simulink model "MIP_LQGcontroller"  (R2020b)
settings: Solver=VariableStepAuto  StartTime=0.0  StopTime=5  RelTol=1e-3
values from neighbouring files (symbols this model uses):
  A = [-(a+b)*j*XX (a+b)*j*XX a*d*XX;(b+c)*j*XX -(b+c)*j*XX -b*d*XX;1 0 0]    [Parameters.m]
  B = [-(a+b)*e*XX; (b+c)*e*XX; 0]    [Parameters.m]
  C = [1 0 0;0 1 0;0 0 1]    [Parameters.m]
  Cy_all = [0 1 0;0 1 0;0 0 1]    [LQG_controller.m]
  Cy_phidot = [0 1 0]    [LQG_controller.m]
  Cy_phidot_theta = [0 1 0;0 0 1]    [LQG_controller.m]
  Cy_theta = [0 0 1]    [LQG_controller.m]
  Cy_thetadot = [1 0 0]    [LQG_controller.m]
  Cy_thetadot_phidot = [1 0 0;0 1 0]    [LQG_controller.m]
  Cy_thetadot_theta = [1 0 0;0 0 1]    [LQG_controller.m]
  D = [0;0;0]    [Parameters.m]
  F_all = -F'    [LQG_controller.m]
  F_phidot = -F'    [LQG_controller.m]
  F_phidot_theta = -F'    [LQG_controller.m]
  F_theta = -F'    [LQG_controller.m]
  F_thetadot = -F'    [LQG_controller.m]
  F_thetadot_phidot = -F'    [LQG_controller.m]
  F_thetadot_theta = -F'    [LQG_controller.m]
  K_all = -K    [LQG_controller.m]
  K_phidot = -K    [LQG_controller.m]
  K_phidot_theta = -K    [LQG_controller.m]
  K_theta = -K    [LQG_controller.m]
  K_thetadot = -K    [LQG_controller.m]
  K_thetadot_phidot = -K    [LQG_controller.m]
  K_thetadot_theta = -K    [LQG_controller.m]
  V_max = 7.4    [Parameters.m]
settings Model: Creator=arthur  LastModifiedBy=arthur

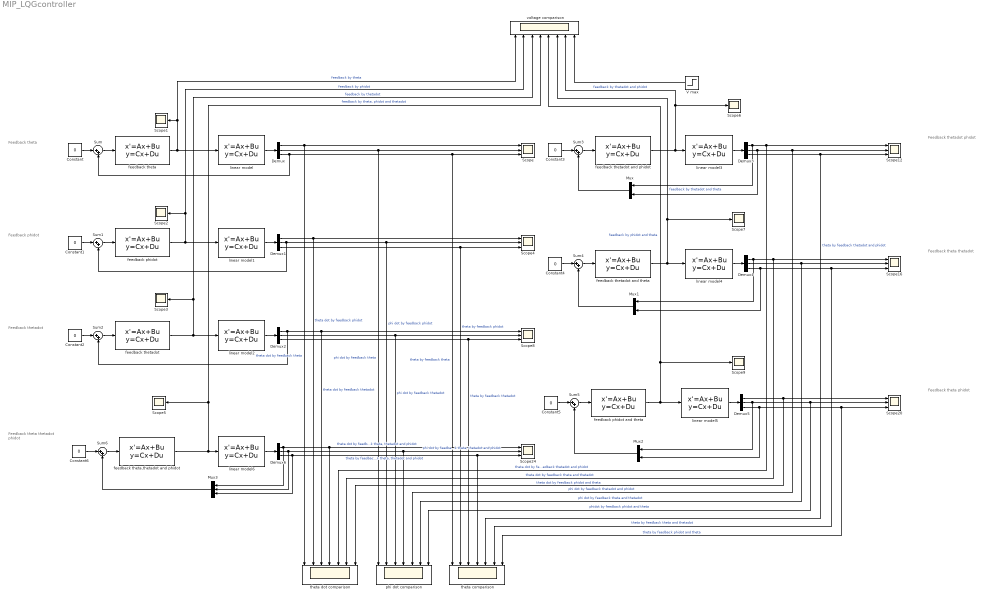
== system MIP_LQGcontroller ==
  note: Feedback
      | theta
  note: Feedback
      | phidot
  note: Feedback
      | thetadot
  note: Feedback
      | theta
      | thetadot
      | phidot
  note: Feedback
      | thetadot
      | phidot
  note: Feedback
      | theta
      | thetadot
  note: Feedback
      | theta
      | phidot
  Constant{,1..6} (7 alike) : Constant  Value=0
  Demux{,1..6} (7 alike) : Demux  Outputs=3
  Mux : Mux  Inputs=2
  Mux1 : Mux  Inputs=2
  Mux2 : Mux  Inputs=2
  Mux3 : Mux  Inputs=3
  Scope{,4,8,12,16,20,24} (7 alike) : Scope  NumInputPorts=3
  Scope{1..3,5..7,9} (7 alike) : Scope
  Sum{,1..6} (7 alike) : Sum  Inputs=|++
  V max : Step  Time=0  After=V_max  SampleTime=0
  feedback phidot : StateSpace  A=A+B*K_phidot+F_phidot*Cy_phidot  B=-F_phidot  C=K_phidot  D=0  InitialCondition=0
  feedback phidot and theta : StateSpace  A=A+B*K_phidot_theta+F_phidot_theta*Cy_phidot_theta  B=-F_phidot_theta  C=K_phidot_theta  D=[0 0]  InitialCondition=0
  feedback theta : StateSpace  A=A+B*K_theta+F_theta*Cy_theta  B=-F_theta  C=K_theta  D=0  InitialCondition=0
  feedback theta,thetadot and phidot : StateSpace  A=A+B*K_all+F_all*Cy_all  B=-F_all  C=K_all  D=[0 0 0]  InitialCondition=0
  feedback thetadot : StateSpace  A=A+B*K_thetadot+F_thetadot*Cy_thetadot  B=-F_thetadot  C=K_thetadot  D=0  InitialCondition=0
  feedback thetadot and phidot : StateSpace  A=A+B*K_thetadot_phidot+F_thetadot_phidot*Cy_thetadot_phidot  B=-F_thetadot_phidot  C=K_thetadot_phidot  D=[0 0]  InitialCondition=0
  feedback thetadot and theta : StateSpace  A=A+B*K_thetadot_theta+F_thetadot_theta*Cy_thetadot_theta  B=-F_thetadot_theta  C=K_thetadot_theta  D=[0 0]  InitialCondition=0
  linear model : StateSpace  A=A  B=B  C=C  D=D  InitialCondition=[0 0 49*pi/180]
  linear model1 : StateSpace  A=A  B=B  C=C  D=D  InitialCondition=[0 0 29*pi/180]
  linear model2 : StateSpace  A=A  B=B  C=C  D=D  InitialCondition=[0 0 30*pi/180]
  linear model3 : StateSpace  A=A  B=B  C=C  D=D  InitialCondition=[0 0 56*pi/180]
  linear model4 : StateSpace  A=A  B=B  C=C  D=D  InitialCondition=[0 0 74*pi/180]
  linear model5 : StateSpace  A=A  B=B  C=C  D=D  InitialCondition=[0 0 48*pi/180]
  linear model6 : StateSpace  A=A  B=B  C=C  D=D  InitialCondition=[0 0 43*pi/180]
  phi dot comparison : Scope  NumInputPorts=7
  theta comparison : Scope  NumInputPorts=7
  theta dot comparison : Scope  NumInputPorts=7
  voltage comparison : Scope  NumInputPorts=8
  wires:
  linear model/1 -> Demux/1
  Demux/1 -> Scope/1, theta dot comparison/1  "theta dot by feedback theta"
  Demux/3 -> Sum/2, Scope/3, theta comparison/1  "theta by feedback theta"
  feedback theta/1 -> linear model/1, Scope1/1, voltage comparison/1  "feedback by theta"
  Demux/2 -> Scope/2, phi dot comparison/1  "phi dot by feedback theta"
  Sum/1 -> feedback theta/1
  Constant/1 -> Sum/1
  feedback phidot/1 -> linear model1/1, Scope2/1, voltage comparison/2  "feedback by phidot"
  Demux1/2 -> Scope4/2, phi dot comparison/2, Sum1/2  "phi dot by feedback phidot"
  Constant1/1 -> Sum1/1
  Sum1/1 -> feedback phidot/1
  Demux1/3 -> Scope4/3, theta comparison/2  "theta by feedback phidot"
  Demux1/1 -> Scope4/1, theta dot comparison/2  "theta dot by feedback phidot"
  linear model1/1 -> Demux1/1
  feedback thetadot/1 -> linear model2/1, Scope3/1, voltage comparison/3  "feedback by thetadot"
  Demux2/2 -> Scope8/2, phi dot comparison/3  "phi dot by feedback thetadot"
  Constant2/1 -> Sum2/1
  Sum2/1 -> feedback thetadot/1
  Demux2/3 -> Scope8/3, theta comparison/3  "theta by feedback thetadot"
  Demux2/1 -> Scope8/1, theta dot comparison/3, Sum2/2  "theta dot by feedback thetadot"
  linear model2/1 -> Demux2/1
  feedback thetadot and phidot/1 -> linear model3/1, Scope6/1, voltage comparison/7  "feedback by thetadot and phidot"
  Demux3/2 -> phi dot comparison/5, Scope12/2, Mux/2  "phi dot by feedback thetadot and phidot"
  Constant3/1 -> Sum3/1
  Sum3/1 -> feedback thetadot and phidot/1
  Demux3/3 -> Scope12/3, theta comparison/5  "theta by feedback thetadot and phidot"
  linear model3/1 -> Demux3/1
  feedback thetadot and theta/1 -> linear model4/1, Scope7/1, voltage comparison/6  "feedback by thetadot and theta"
  Demux4/2 -> Scope16/2, phi dot comparison/6  "phi dot by feedback theta and thetadot"
  Constant4/1 -> Sum4/1
  Sum4/1 -> feedback thetadot and theta/1
  Demux4/1 -> Scope16/1, theta dot comparison/6, Mux1/1  "theta dot by feedback theta and thetadot"
  linear model4/1 -> Demux4/1
  feedback phidot and theta/1 -> linear model5/1, voltage comparison/5, Scope9/1  "feedback by phidot and theta"
  Demux5/2 -> Scope20/2, phi dot comparison/7, Mux2/1  "phidot by feedback phidot and theta"
  Constant5/1 -> Sum5/1
  Sum5/1 -> feedback phidot and theta/1
  Demux5/3 -> Scope20/3, theta comparison/7, Mux2/2  "theta by feedback phidot and theta"
  Demux5/1 -> Scope20/1, theta dot comparison/7  "theta dot by feedback phidot and theta"
  linear model5/1 -> Demux5/1
  feedback theta,thetadot and phidot/1 -> linear model6/1, Scope5/1, voltage comparison/4  "feedback by theta, phidot and thetadot"
  Demux6/2 -> Scope24/2, phi dot comparison/4, Mux3/2  "phi dot by feedback theta, thetadot and phidot"
  Constant6/1 -> Sum6/1
  Sum6/1 -> feedback theta,thetadot and phidot/1
  Demux6/3 -> Scope24/3, theta comparison/4, Mux3/3  "theta by feedback theta, thetadot and phidot"
  Demux6/1 -> Scope24/1, theta dot comparison/4, Mux3/1  "theta dot by feedback theta, thetadot and phidot"
  linear model6/1 -> Demux6/1
  Mux/1 -> Sum3/2
  Mux1/1 -> Sum4/2
  Demux4/3 -> Scope16/3, theta comparison/6, Mux1/2  "theta by feedback theta and thetadot"
  Mux2/1 -> Sum5/2
  Mux3/1 -> Sum6/2
  Demux3/1 -> Scope12/1, theta dot comparison/5, Mux/1  "theta dot by feedback thetadot and phidot"
  V max/1 -> voltage comparison/8
